simulink model "task_2_sim"  (R2022b)
settings: Solver=VariableStepAuto  StartTime=0.0  StopTime=10.0  RelTol=1e-3
values from neighbouring files (symbols this model uses):
  K2_1 = getLQRController(A, B, Q, R)    [task2.m]
undefined symbols (not defined in the file or in its folder): A, B, C
settings Model: Creator=小灰  LastModifiedBy=小灰

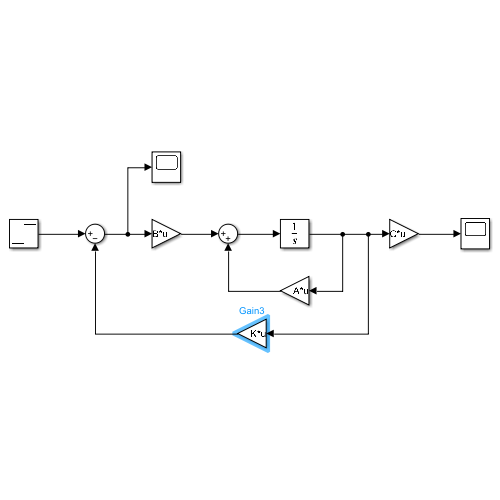
[thumbnail: Simulink's stored preview of the top-level diagram]
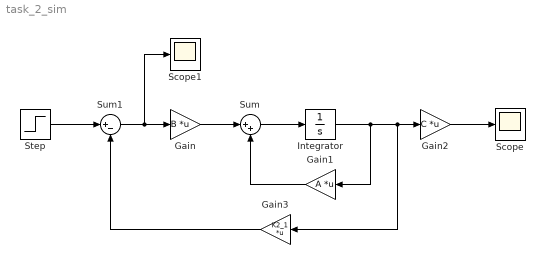
== system task_2_sim ==
  Gain : Gain  Gain=B  Multiplication=Matrix(K*u)
  Gain1 : Gain  Gain=A  Multiplication=Matrix(K*u)
  Gain2 : Gain  Gain=C  Multiplication=Matrix(K*u)
  Gain3 : Gain  Gain=K2_1  Multiplication=Matrix(K*u)
  Integrator : Integrator
  Scope : Scope
  Scope1 : Scope
  Step : Step  SampleTime=0
  Sum : Sum  Inputs=|++
  Sum1 : Sum  Inputs=|+-
  wires:
  Integrator/1 -> Gain1/1, Gain3/1, Gain2/1
  Sum/1 -> Integrator/1
  Step/1 -> Sum1/1
  Gain2/1 -> Scope/1
  Gain1/1 -> Sum/2
  Sum1/1 -> Scope1/1, Gain/1
  Gain/1 -> Sum/1
  Gain3/1 -> Sum1/2
